simulink model "Planta_Seguimiento_Integrador"  (R2021a)
settings: Solver=FixedStepAuto  StartTime=0.0  StopTime=5  FixedStep=0.001  RelTol=1e-3
values from neighbouring files (symbols this model uses):
  A = [0 0 0 1;0 1446.9 213.6 -57.9;0 1 0 0;0 -126.3 -12.8 5.1]    [1_DiseñoRegulador_Seguidor_Discreto.m]    (also in Control_Seguimiento_Integrador_MATLAB.m = [0,1,0,0;0,-0.221772837618740,0.450086090591265,-0.661704776; Controlador.m = [0 1 0 0;0 -6.109*10^(-08)   2.828*10^(-5)  -7.749*10^(-6);0; Leo_Controlador.m = [0,1,0,0;0,-18.1491205715699,-0.241940259070541,-0.001617883; funcmotor.m = [0 1 0 0;0 par(1) par(2) par(3);0 0 0 1;0 par(4) par(5) par()
  B = [0;-122.6;0;10.7]    [1_DiseñoRegulador_Seguidor_Discreto.m]    (also in Control_Seguimiento_Integrador_MATLAB.m = [0;1.02819574469726;0;2.93672730148517]; Controlador.m = [0;-2.126*10^(-8);0;-293]; Leo_Controlador.m = [0;3.24704785577389;0;142.313463961677]; funcmotor.m = [0;par(7);0;par(8)])
  K1 = acker(Aa,Ba,raices2)    [Control_Seguimiento_Integrador_MATLAB.m]
undefined symbols (not defined in the file or in its folder): DiscIntNeverNeededParam
settings Model: Creator=diego  LastModifiedBy=Sinso

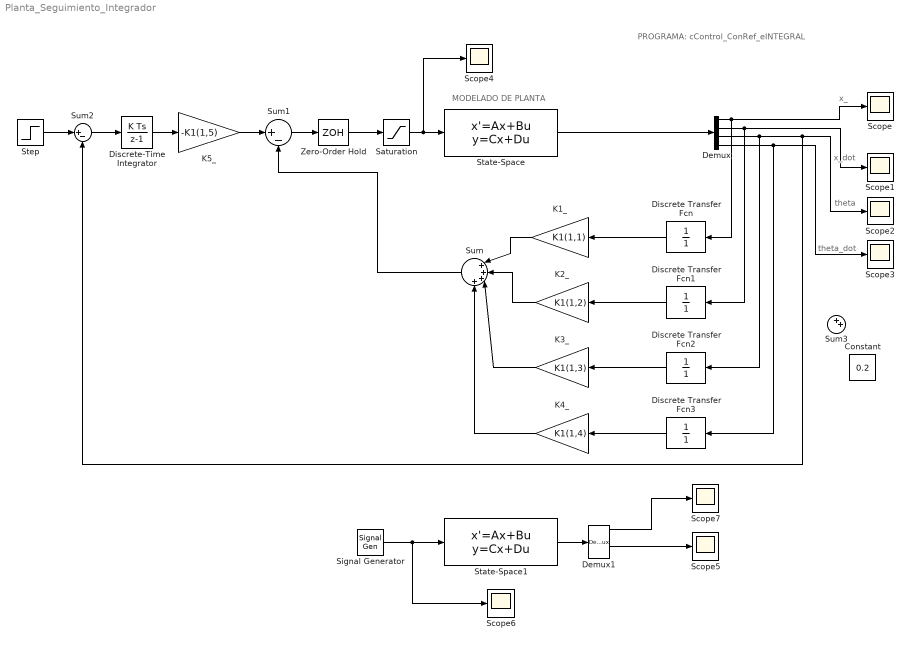
== system Planta_Seguimiento_Integrador ==
  note: theta_dot
  note: theta
  note: x_dot
  note: x_
  note: MODELADO DE PLANTA
  note: PROGRAMA: cControl_ConRef_eINTEGRAL
  Constant : Constant  Value=0.2
  Demux : Demux
  Demux1 : Demux
  Discrete Transfer Fcn{,1..3} (4 alike) : DiscreteTransferFcn  Denominator=[1 ]  SampleTime=0.001
  Discrete-Time Integrator : DiscreteIntegrator  SampleTime=0.001  ICPrevOutput=DiscIntNeverNeededParam  ICPrevScaledInput=DiscIntNeverNeededParam
  K1_ : Gain  Gain=K1(1,1)
  K2_ : Gain  Gain=K1(1,2)
  K3_ : Gain  Gain=K1(1,3)
  K4_ : Gain  Gain=K1(1,4)
  K5_ : Gain  Gain=-K1(1,5)
  Saturation : Saturate  UpperLimit=5  LowerLimit=-5
  Scope{,1..7} (8 alike) : Scope
  Signal Generator : SignalGenerator  WaveForm=square  Amplitude=2.5  Frequency=10
  State-Space : StateSpace  A=A  B=B  C=[1 0 0 0;0 1 0 0; 0 0 1 0; 0 0 0 1]  D=[0;0;0;0]  InitialCondition=0
  State-Space1 : StateSpace  A=A  B=B  C=[1 0 0 0;0 1 0 0; 0 0 1 0; 0 0 0 1]  D=[0;0;0;0]  InitialCondition=0
  Step : Step  After=0  SampleTime=0
  Sum : Sum  Inputs=|++++
  Sum1 : Sum  Inputs=|+-
  Sum2 : Sum  Inputs=|+-
  Sum3 : Sum  Inputs=|++
  Zero-Order Hold : ZeroOrderHold  SampleTime=0.001
  wires:
  Sum2/1 -> Discrete-Time Integrator/1
  Discrete-Time Integrator/1 -> K5_/1
  Step/1 -> Sum2/1
  Sum1/1 -> Zero-Order Hold/1
  Zero-Order Hold/1 -> Saturation/1
  State-Space/1 -> Demux/1
  Demux/2 -> Discrete Transfer Fcn1/1, Scope1/1
  Demux/3 -> Sum2/2, Scope2/1, Discrete Transfer Fcn2/1
  Demux/4 -> Discrete Transfer Fcn3/1, Scope3/1
  K1_/1 -> Sum/1
  K2_/1 -> Sum/2
  K3_/1 -> Sum/3
  K4_/1 -> Sum/4
  Sum/1 -> Sum1/2
  K5_/1 -> Sum1/1
  Demux/1 -> Discrete Transfer Fcn/1, Scope/1
  Discrete Transfer Fcn/1 -> K1_/1
  Discrete Transfer Fcn1/1 -> K2_/1
  Discrete Transfer Fcn2/1 -> K3_/1
  Discrete Transfer Fcn3/1 -> K4_/1
  Saturation/1 -> Scope4/1, State-Space/1
  Signal Generator/1 -> Scope6/1, State-Space1/1
  State-Space1/1 -> Demux1/1
  Demux1/3 -> Scope5/1
  Demux1/1 -> Scope7/1
